simulink library "VLS_Standard_Library"  (R2017b)
settings: Solver=VariableStepAuto  StartTime=0.0  StopTime=10.0  RelTol=1e-3
libraries: simulink x10
Description:
  | VLS Standard Library
  | Version: 1.0.1
settings Model: Creator=mchawa  LastModifiedBy=mchawa

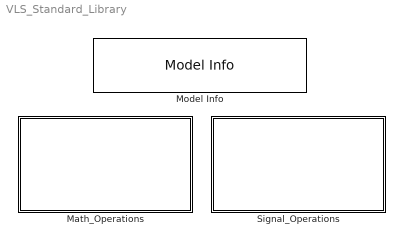
== system VLS_Standard_Library ==
  Math_Operations : Subsystem
  Model Info : simulink/Model-Wide Utilities/Model Info  Frame=on  DisplayStringWithTags=|  HorizontalTextAlignment=Center  LeftAlignmentValue=0.5
      | Model Info
      | Name: %<ModelName>
      | Description: %<Description>
  Signal_Operations : Subsystem

== system VLS_Standard_Library/Math_Operations ==
  SimpleSecureDivision : Subsystem

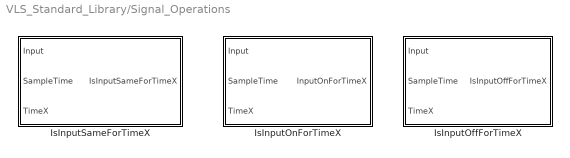
== system VLS_Standard_Library/Signal_Operations ==
  IsInputOffForTimeX : Subsystem
  IsInputOnForTimeX : Subsystem
  IsInputSameForTimeX : Subsystem

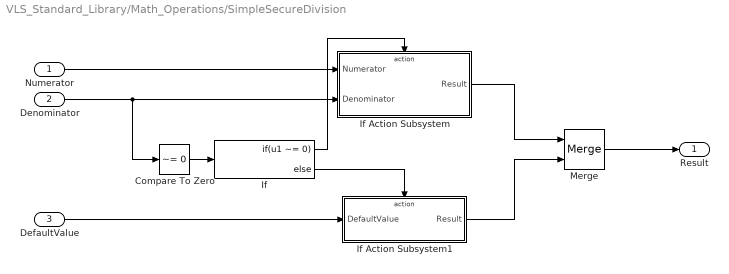
== system VLS_Standard_Library/Math_Operations/SimpleSecureDivision ==
  Numerator : Inport
  Denominator : Inport  Port=2
  DefaultValue : Inport  Port=3
  Compare To Zero : simulink/Logic and Bit Operations/Compare To Zero  relop=~=  OutDataTypeStr=boolean
  If : If  IfExpression=u1 ~= 0
  If Action Subsystem : Subsystem  TreatAsAtomicUnit=on
  If Action Subsystem1 : Subsystem  TreatAsAtomicUnit=on
  Merge : Merge
  Result : Outport
  wires:
  Numerator/1 -> If Action Subsystem/1(Numerator)
  If/2 -> If Action Subsystem1/Action
  Denominator/1 -> If Action Subsystem/2(Denominator), Compare To Zero/1
  If Action Subsystem/1(Result) -> Merge/1
  If Action Subsystem1/1(Result) -> Merge/2
  Merge/1 -> Result/1
  DefaultValue/1 -> If Action Subsystem1/1(DefaultValue)
  If/1 -> If Action Subsystem/Action
  Compare To Zero/1 -> If/1

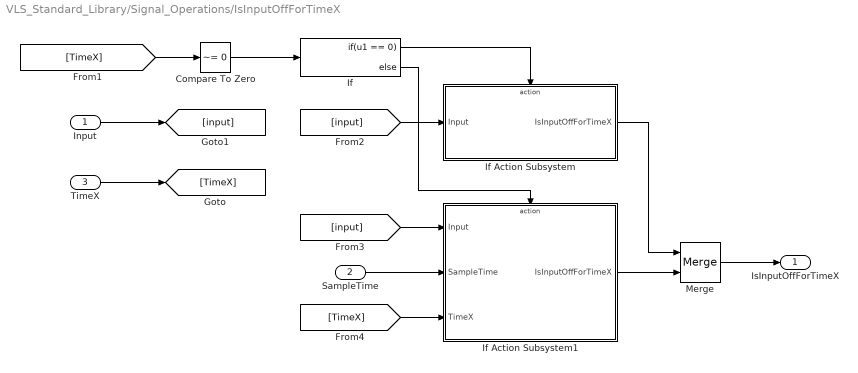
== system VLS_Standard_Library/Signal_Operations/IsInputOffForTimeX ==
  Input : Inport
  SampleTime : Inport  Port=2
  TimeX : Inport  Port=3
  Compare To Zero : simulink/Logic and Bit Operations/Compare To Zero  relop=~=  OutDataTypeStr=boolean
  If : If  IfExpression=u1 == 0
  If Action Subsystem : Subsystem  TreatAsAtomicUnit=on
  If Action Subsystem1 : Subsystem  TreatAsAtomicUnit=on
  Merge : Merge
  IsInputOffForTimeX : Outport
  wires:
  Compare To Zero/1 -> If/1
  Merge/1 -> IsInputOffForTimeX/1
  If Action Subsystem1/1(IsInputOffForTimeX) -> Merge/2
  If Action Subsystem/1(IsInputOffForTimeX) -> Merge/1
  [TimeX] -> If Action Subsystem1/3(TimeX)
  [TimeX] -> Compare To Zero/1
  TimeX/1 -> [TimeX]
  If/2 -> If Action Subsystem1/Action
  SampleTime/1 -> If Action Subsystem1/2(SampleTime)
  [input] -> If Action Subsystem1/1(Input)
  [input] -> If Action Subsystem/1(Input)
  Input/1 -> [input]
  If/1 -> If Action Subsystem/Action

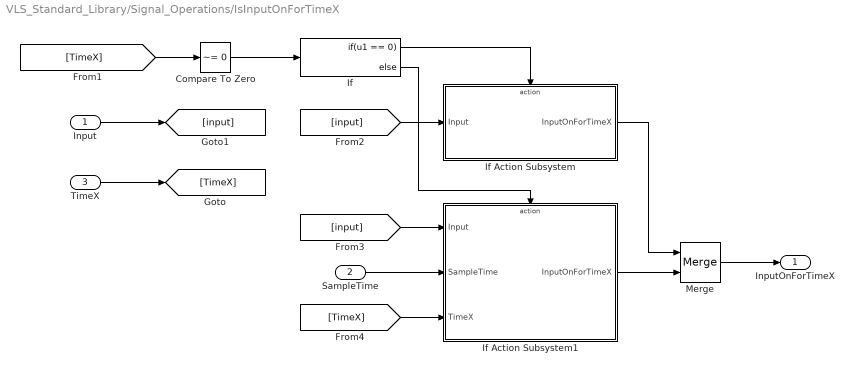
== system VLS_Standard_Library/Signal_Operations/IsInputOnForTimeX ==
  Input : Inport
  SampleTime : Inport  Port=2
  TimeX : Inport  Port=3
  Compare To Zero : simulink/Logic and Bit Operations/Compare To Zero  relop=~=  OutDataTypeStr=boolean
  If : If  IfExpression=u1 == 0
  If Action Subsystem : Subsystem  TreatAsAtomicUnit=on
  If Action Subsystem1 : Subsystem  TreatAsAtomicUnit=on
  Merge : Merge
  InputOnForTimeX : Outport
  wires:
  If/1 -> If Action Subsystem/Action
  Input/1 -> [input]
  [input] -> If Action Subsystem/1(Input)
  [input] -> If Action Subsystem1/1(Input)
  SampleTime/1 -> If Action Subsystem1/2(SampleTime)
  If/2 -> If Action Subsystem1/Action
  TimeX/1 -> [TimeX]
  [TimeX] -> Compare To Zero/1
  [TimeX] -> If Action Subsystem1/3(TimeX)
  If Action Subsystem/1(InputOnForTimeX) -> Merge/1
  If Action Subsystem1/1(InputOnForTimeX) -> Merge/2
  Merge/1 -> InputOnForTimeX/1
  Compare To Zero/1 -> If/1

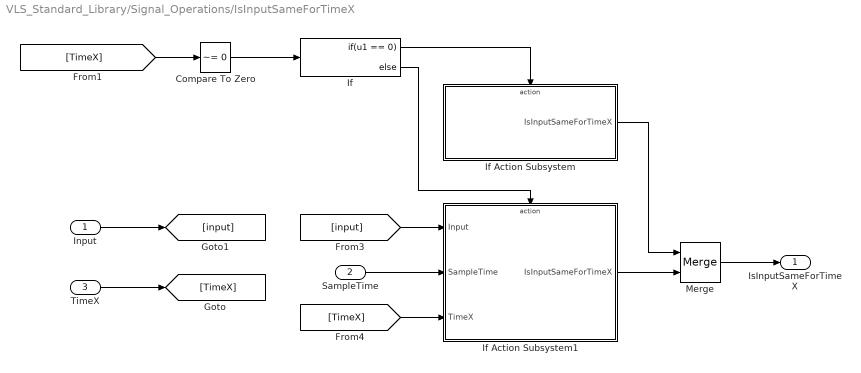
== system VLS_Standard_Library/Signal_Operations/IsInputSameForTimeX ==
  Input : Inport
  SampleTime : Inport  Port=2
  TimeX : Inport  Port=3
  Compare To Zero : simulink/Logic and Bit Operations/Compare To Zero  relop=~=  OutDataTypeStr=boolean
  If : If  IfExpression=u1 == 0
  If Action Subsystem : Subsystem  TreatAsAtomicUnit=on
  If Action Subsystem1 : Subsystem  TreatAsAtomicUnit=on
  Merge : Merge
  IsInputSameForTimeX : Outport
  wires:
  Compare To Zero/1 -> If/1
  Merge/1 -> IsInputSameForTimeX/1
  If Action Subsystem1/1(IsInputSameForTimeX) -> Merge/2
  If Action Subsystem/1(IsInputSameForTimeX) -> Merge/1
  [TimeX] -> If Action Subsystem1/3(TimeX)
  [TimeX] -> Compare To Zero/1
  TimeX/1 -> [TimeX]
  If/2 -> If Action Subsystem1/Action
  SampleTime/1 -> If Action Subsystem1/2(SampleTime)
  [input] -> If Action Subsystem1/1(Input)
  Input/1 -> [input]
  If/1 -> If Action Subsystem/Action

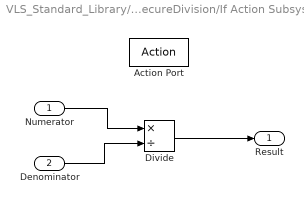
== system VLS_Standard_Library/Math_Operations/SimpleSecureDivision/If Action Subsystem ==
  Numerator : Inport
  Denominator : Inport  Port=2
  Action Port : ActionPort
  Divide : Product  Inputs=*/  OutDataTypeStr=Inherit: Inherit via back propagation
  Result : Outport
  wires:
  Divide/1 -> Result/1
  Numerator/1 -> Divide/1
  Denominator/1 -> Divide/2

== system VLS_Standard_Library/Math_Operations/SimpleSecureDivision/If Action Subsystem1 ==
  DefaultValue : Inport
  Action Port : ActionPort
  Result : Outport
  wires:
  DefaultValue/1 -> Result/1

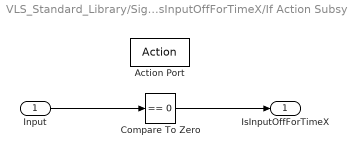
== system VLS_Standard_Library/Signal_Operations/IsInputOffForTimeX/If Action Subsystem ==
  Input : Inport
  Action Port : ActionPort
  Compare To Zero : simulink/Logic and Bit Operations/Compare To Zero  relop===  OutDataTypeStr=boolean
  IsInputOffForTimeX : Outport
  wires:
  Compare To Zero/1 -> IsInputOffForTimeX/1
  Input/1 -> Compare To Zero/1

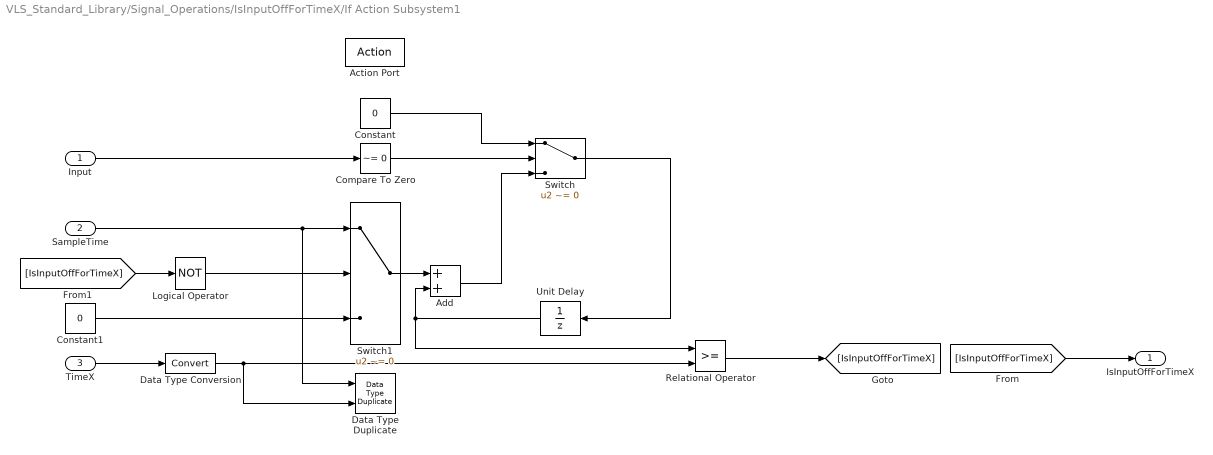
== system VLS_Standard_Library/Signal_Operations/IsInputOffForTimeX/If Action Subsystem1 ==
  Input : Inport
  SampleTime : Inport  Port=2
  TimeX : Inport  Port=3
  Action Port : ActionPort
  Add : Sum
  Compare To Zero : simulink/Logic and Bit Operations/Compare To Zero  relop=~=  OutDataTypeStr=boolean
  Constant : Constant  Value=0  OutDataTypeStr=Inherit: Inherit via back propagation
  Constant1 : Constant  Value=0  OutDataTypeStr=Inherit: Inherit via back propagation
  Data Type Duplicate : DataTypeDuplicate
  Data Type Conversion : DataTypeConversion  SaturateOnIntegerOverflow=on
  Logical Operator : Logic  Operator=NOT  AllPortsSameDT=off  OutDataTypeStr=boolean
  Relational Operator : RelationalOperator  OutDataTypeStr=boolean  RndMeth=Simplest
  Switch : Switch  Criteria=u2 ~= 0
  Switch1 : Switch  Criteria=u2 ~= 0
  Unit Delay : UnitDelay  SampleTime=-1
  IsInputOffForTimeX : Outport
  wires:
  TimeX/1 -> Data Type Conversion/1
  Input/1 -> Compare To Zero/1
  Unit Delay/1 -> Add/2, Relational Operator/1
  Constant/1 -> Switch/1
  Compare To Zero/1 -> Switch/2
  Add/1 -> Switch/3
  Switch/1 -> Unit Delay/1
  Switch1/1 -> Add/1
  SampleTime/1 -> Switch1/1, Data Type Duplicate/1
  Logical Operator/1 -> Switch1/2
  Constant1/1 -> Switch1/3
  [IsInputOffForTimeX] -> IsInputOffForTimeX/1
  Data Type Conversion/1 -> Relational Operator/2, Data Type Duplicate/2
  [IsInputOffForTimeX] -> Logical Operator/1
  Relational Operator/1 -> [IsInputOffForTimeX]

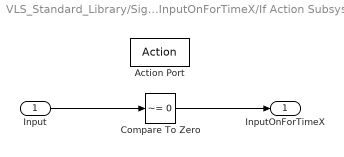
== system VLS_Standard_Library/Signal_Operations/IsInputOnForTimeX/If Action Subsystem ==
  Input : Inport
  Action Port : ActionPort  ActionType=then
  Compare To Zero : simulink/Logic and Bit Operations/Compare To Zero  relop=~=  OutDataTypeStr=boolean
  InputOnForTimeX : Outport
  wires:
  Input/1 -> Compare To Zero/1
  Compare To Zero/1 -> InputOnForTimeX/1

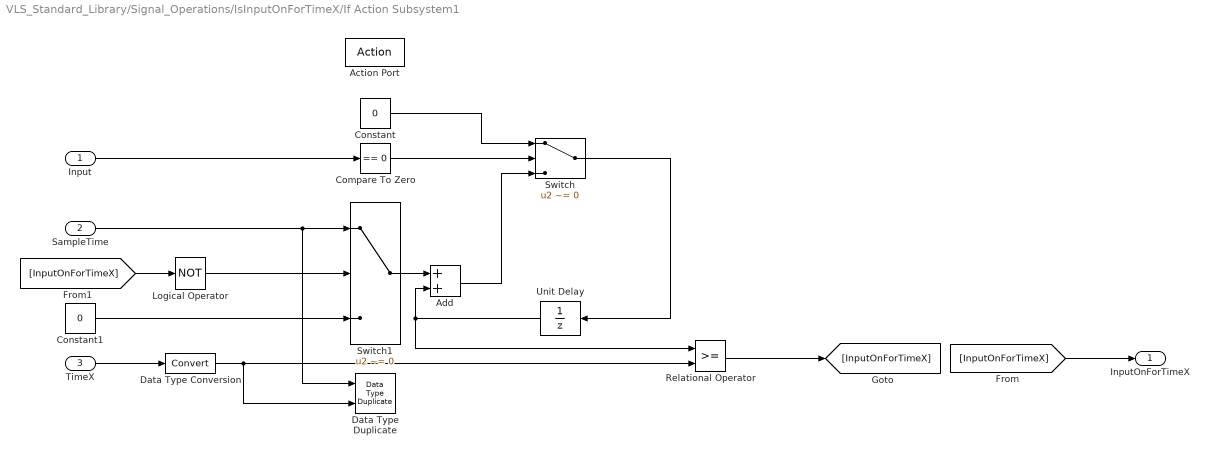
== system VLS_Standard_Library/Signal_Operations/IsInputOnForTimeX/If Action Subsystem1 ==
  Input : Inport
  SampleTime : Inport  Port=2
  TimeX : Inport  Port=3
  Action Port : ActionPort  ActionType=else
  Add : Sum
  Compare To Zero : simulink/Logic and Bit Operations/Compare To Zero  relop===  OutDataTypeStr=boolean
  Constant : Constant  Value=0  OutDataTypeStr=Inherit: Inherit via back propagation
  Constant1 : Constant  Value=0  OutDataTypeStr=Inherit: Inherit via back propagation
  Data Type Duplicate : DataTypeDuplicate
  Data Type Conversion : DataTypeConversion  SaturateOnIntegerOverflow=on
  Logical Operator : Logic  Operator=NOT  AllPortsSameDT=off  OutDataTypeStr=boolean
  Relational Operator : RelationalOperator  OutDataTypeStr=boolean  RndMeth=Simplest
  Switch : Switch  Criteria=u2 ~= 0
  Switch1 : Switch  Criteria=u2 ~= 0
  Unit Delay : UnitDelay  SampleTime=-1
  InputOnForTimeX : Outport
  wires:
  Relational Operator/1 -> [InputOnForTimeX]
  [InputOnForTimeX] -> Logical Operator/1
  Data Type Conversion/1 -> Data Type Duplicate/2, Relational Operator/2
  [InputOnForTimeX] -> InputOnForTimeX/1
  Constant1/1 -> Switch1/3
  Logical Operator/1 -> Switch1/2
  SampleTime/1 -> Data Type Duplicate/1, Switch1/1
  Switch1/1 -> Add/1
  Switch/1 -> Unit Delay/1
  Add/1 -> Switch/3
  Compare To Zero/1 -> Switch/2
  Constant/1 -> Switch/1
  Unit Delay/1 -> Relational Operator/1, Add/2
  Input/1 -> Compare To Zero/1
  TimeX/1 -> Data Type Conversion/1

== system VLS_Standard_Library/Signal_Operations/IsInputSameForTimeX/If Action Subsystem ==
  Action Port : ActionPort
  Constant : Constant  Value=true  OutDataTypeStr=boolean
  IsInputSameForTimeX : Outport
  wires:
  Constant/1 -> IsInputSameForTimeX/1

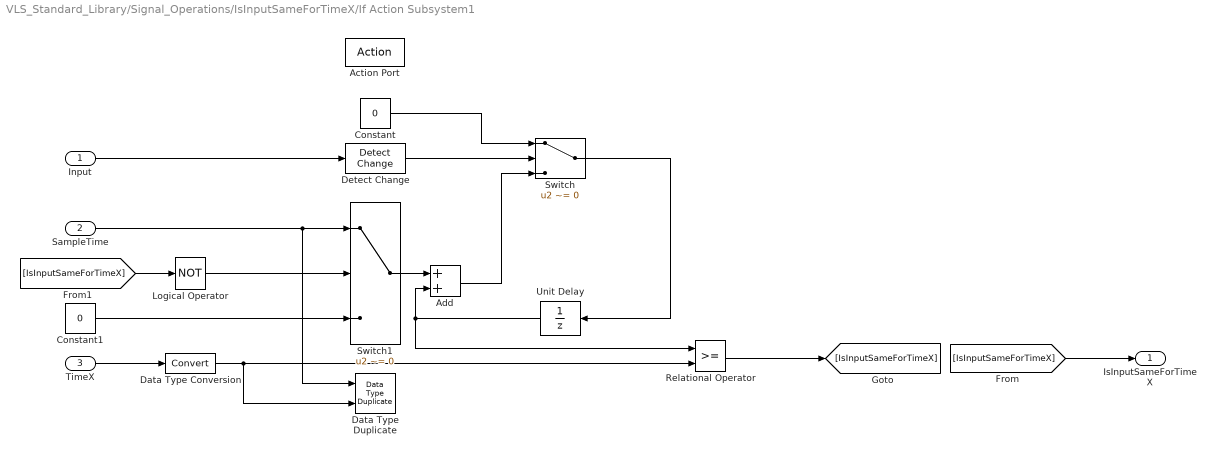
== system VLS_Standard_Library/Signal_Operations/IsInputSameForTimeX/If Action Subsystem1 ==
  Input : Inport
  SampleTime : Inport  Port=2
  TimeX : Inport  Port=3
  Action Port : ActionPort
  Add : Sum
  Constant : Constant  Value=0  OutDataTypeStr=Inherit: Inherit via back propagation
  Constant1 : Constant  Value=0  OutDataTypeStr=Inherit: Inherit via back propagation
  Data Type Duplicate : DataTypeDuplicate
  Data Type Conversion : DataTypeConversion  SaturateOnIntegerOverflow=on
  Detect Change : simulink/Logic and Bit Operations/Detect Change  vinit=0  OutDataTypeStr=boolean
  Logical Operator : Logic  Operator=NOT  AllPortsSameDT=off  OutDataTypeStr=boolean
  Relational Operator : RelationalOperator  OutDataTypeStr=boolean  RndMeth=Simplest
  Switch : Switch  Criteria=u2 ~= 0
  Switch1 : Switch  Criteria=u2 ~= 0
  Unit Delay : UnitDelay  SampleTime=-1
  IsInputSameForTimeX : Outport
  wires:
  TimeX/1 -> Data Type Conversion/1
  Input/1 -> Detect Change/1
  Unit Delay/1 -> Add/2, Relational Operator/1
  Constant/1 -> Switch/1
  Detect Change/1 -> Switch/2
  Add/1 -> Switch/3
  Switch/1 -> Unit Delay/1
  Switch1/1 -> Add/1
  SampleTime/1 -> Switch1/1, Data Type Duplicate/1
  Logical Operator/1 -> Switch1/2
  Constant1/1 -> Switch1/3
  [IsInputSameForTimeX] -> IsInputSameForTimeX/1
  Data Type Conversion/1 -> Relational Operator/2, Data Type Duplicate/2
  [IsInputSameForTimeX] -> Logical Operator/1
  Relational Operator/1 -> [IsInputSameForTimeX]
